simulink model "ModeLogicModule"  (R2020a)
settings: configuration reference "SLRT" (kept outside this file)
settings Model: DataDictionary=SGKitControllerData.sldd  EnableAccessToBaseWorkspace=off  Creator=The MathWorks, Inc.  LastModifiedBy=daniel.fonte
settings ConfigSetRef: SourceName=SLRT

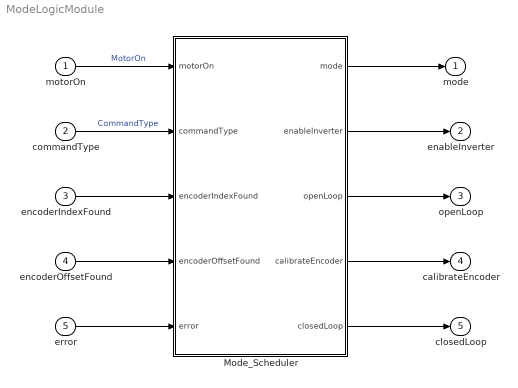
== system ModeLogicModule ==
  motorOn : Inport  OutDataTypeStr=boolean  PortDimensions=1  SampleTime=[0.001,0]
  commandType : Inport  Port=2  OutDataTypeStr=Enum: commandTypeEnum  PortDimensions=1  SampleTime=[0.001,0]
  encoderIndexFound : Inport  Port=3  OutDataTypeStr=boolean  PortDimensions=1  SampleTime=[0.001,0]
  encoderOffsetFound : Inport  Port=4  OutDataTypeStr=boolean  PortDimensions=1  SampleTime=[0.001,0]
  error : Inport  Port=5  OutDataTypeStr=boolean  PortDimensions=1  SampleTime=[0.001,0]
  Mode_Scheduler : Stateflow chart  TreatAsAtomicUnit=on
  mode : Outport  OutDataTypeStr=Enum: modeSchedulerEnum  PortDimensions=1  SampleTime=[0.001,0]  VectorParamsAs1DForOutWhenUnconnected=off
  " enableInverter" : Outport  Port=2  OutDataTypeStr=boolean  PortDimensions=1  SampleTime=[0.001,0]  VectorParamsAs1DForOutWhenUnconnected=off
  " openLoop" : Outport  Port=3  OutDataTypeStr=boolean  PortDimensions=1  SampleTime=[0.001,0]  VectorParamsAs1DForOutWhenUnconnected=off
  " calibrateEncoder" : Outport  Port=4  OutDataTypeStr=boolean  PortDimensions=1  SampleTime=[0.001,0]  VectorParamsAs1DForOutWhenUnconnected=off
  " closedLoop" : Outport  Port=5  OutDataTypeStr=boolean  PortDimensions=1  SampleTime=[0.001,0]  VectorParamsAs1DForOutWhenUnconnected=off
  wires:
  motorOn/1 -> Mode_Scheduler/1(motorOn)  "MotorOn"
  commandType/1 -> Mode_Scheduler/2(commandType)  "CommandType"
  encoderIndexFound/1 -> Mode_Scheduler/3(encoderIndexFound)
  encoderOffsetFound/1 -> Mode_Scheduler/4(encoderOffsetFound)
  error/1 -> Mode_Scheduler/5(error)
  Mode_Scheduler/1(mode) -> mode/1
  Mode_Scheduler/2(" enableInverter") -> " enableInverter"/1
  Mode_Scheduler/3(" openLoop") -> " openLoop"/1
  Mode_Scheduler/4(" calibrateEncoder") -> " calibrateEncoder"/1
  Mode_Scheduler/5(" closedLoop") -> " closedLoop"/1

== stateflow chart ModeLogicModule/Mode_Scheduler ==
  settings: updateMethod=DISCRETE
  note: Mode Scheduler
  state Enable_Inverter
    state Open_Loop
      state Open_Loop_Command
      state Find_Encoder_Index
    state Calibrate_Encoder_Offset
    state Closed_Loop
    (junction 378) -> Open_Loop_Command [order 1] : [commandType == ...
        |  commandTypeEnum.OpenLoopVelocity]
    (junction 378) -> (junction 624) [order 2]
    Open_Loop_Command -> (junction 624) : [commandType ~= ...
        |  commandTypeEnum.OpenLoopVelocity]
    (junction 624) -> (junction 619)
    (junction 619) -> (junction 638) [order 1] : [(commandType == ...
        |   commandTypeEnum.CalibrateEncoder) ...
        |  || (paramEncoderCalibrateAtStartup ...
        |      && ~encoderOffsetFound) ]
    (junction 638) -> Find_Encoder_Index [order 1] : [~encoderIndexFound]
    (junction 638) -> (junction 640) [order 2]
    (junction 619) -> (junction 604) [order 2]
    Find_Encoder_Index -> Calibrate_Encoder_Offset : [encoderIndexFound]
    (junction 640) -> Calibrate_Encoder_Offset
    Calibrate_Encoder_Offset -> (junction 604) : [(commandType ~= ...
        |   commandTypeEnum.CalibrateEncoder) ...
        |   && encoderOffsetFound]
    (junction 604) -> (junction 232)
    (junction 232) -> Closed_Loop [order 1] : [commandType == ...
        |  commandTypeEnum.Velocity]
    (junction 232) -> (junction 627) [order 2]
    Closed_Loop -> (junction 627) : [commandType ~= ...
        |  commandTypeEnum.Velocity]
  state Stand_By
  state Error
  (default) -> Stand_By
  Stand_By -> (junction 378) : [motorOn]
  Enable_Inverter -> Stand_By [order 1] : [~motorOn]
  Error -> Stand_By : [~motorOn]
  Enable_Inverter -> Error [order 2] : [error]
  (junction 627) -> Error
  data: mode output Enum: modeSchedulerEnum; enableInverter output boolean; motorOn input; commandType input; encoderIndexFound input; openLoop output boolean; calibrateEncoder output boolean; closedLoop output boolean; encoderOffsetFound input; error input; paramEncoderCalibrateAtStartup parameter boolean
